simulink subsystem "ControladorBA"  (R2023b)
settings: Solver=VariableStepAuto  StartTime=0.0  StopTime=10.0  RelTol=1e-3
settings Model: Creator=johan  LastModifiedBy=Carlos

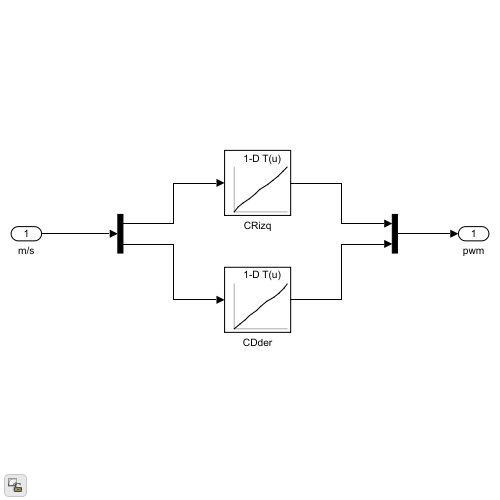
[thumbnail: Simulink's stored preview of the top-level diagram]
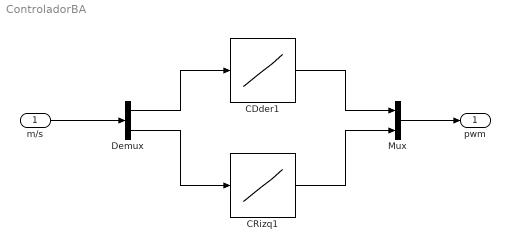
== system ControladorBA ==
  m/s : Inport
  CDder1 : Lookup_n-D  NumberOfTableDimensions=1  BreakpointsForDimension1=[-0.486428320407867 -0.378355830907822 -0.283766865730286 -0.202680960297585 -0.0810762494802475 0 0.10809651017189 0.229699119925499 0.324297249317169 0.418877989053726 0.472927540540695]  Table=[-255 -200 -150 -100 -50 0 50 100 150 200 255]  InternalRulePriority=Speed  RndMeth=Simplest
  CRizq1 : Lookup_n-D  NumberOfTableDimensions=1  BreakpointsForDimension1=[-0.486428320407867 -0.405375272035599 -0.310786336660385 -0.202674999833107 -0.0810762494802475 0 0.135120630264282 0.229705080389977 0.337809652090073 0.43239039182663 0.49995231628418]  Table=[-255 -200 -150 -100 -50 0 50 100 150 200 255]  InternalRulePriority=Speed  RndMeth=Simplest
  Demux : Demux  Outputs=2
  Mux : Mux  Inputs=2
  pwm : Outport
  wires:
  CDder1/1 -> Mux/1
  CRizq1/1 -> Mux/2
  Demux/2 -> CRizq1/1
  Demux/1 -> CDder1/1
  m/s/1 -> Demux/1
  Mux/1 -> pwm/1
